simulink model "fourtankssim"  (Simulink 5.1)
settings: Solver=ode45  StartTime=0.0  StopTime=1000  RelTol=1e-3
libraries: mpt_sim x2
settings Model: LastModifiedBy=michal  BooleanDataType=on

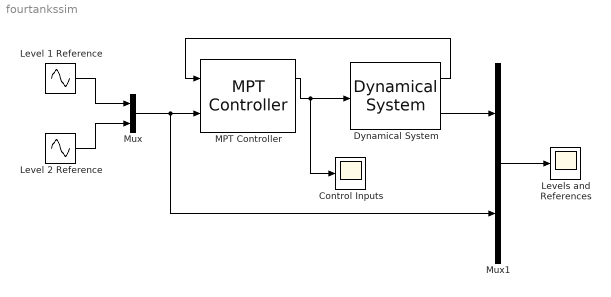
== system fourtankssim ==
  Control Inputs : Scope
      settings: TimeRange=1000  YMin=-1  YMax=1  SaveToWorkspace=off  LimitDataPoints=on  MaxDataPoints=5000
  Dynamical System : mpt_sim/Dynamical System  sysStruct=sysStruct  x0=[0;0;0;0]  Ts=[]  constr=on
  Level 1 Reference : Sin  Amplitude=2  Frequency=0.01  Phase=0  SampleTime=0
  Level 2 Reference : Sin  Amplitude=1  Frequency=0.01  Phase=1  SampleTime=0
  Levels and References : Scope
      settings: TimeRange=1000  YMin=-3  YMax=3  SaveToWorkspace=off  SaveName=ScopeData  LimitDataPoints=on  MaxDataPoints=5000
  MPT Controller : mpt_sim/MPT Controller  ctrl=onlinec  Ts=[]  infbreak=on
  Mux : Mux  Inputs=2
  Mux1 : Mux  Inputs=2
  wires:
  Level 1 Reference/1 -> Mux/1
  Level 2 Reference/1 -> Mux/2
  Mux/1 -> MPT Controller/2, Mux1/2
  MPT Controller/1 -> Dynamical System/1, Control Inputs/1
  Dynamical System/1 -> MPT Controller/1
  Dynamical System/2 -> Mux1/1
  Mux1/1 -> Levels and References/1
